simulink model "acc_with_sensor"  (R2021b)
settings: Solver=FixedStepAuto  StartTime=0.0  StopTime=206  FixedStep=0.0005  RelTol=1e-3
InitFcn:
  | G=9.81;
  | m=1660;
  | rw=0.325;
  | Caf=74070;
  | Car=58525;
  | Iz=2778.5;
  | d = 1.502;
  | lf =1.1135;
  | lr =1.5065;
  | L = 2.62;
  | kph2mps=1/3.6;
values from neighbouring files (symbols this model uses):
  Leftdis_PV_switch = 2    [acc_plot_backup.m]
  s_path = [0 1.10508939428 2.2141958029 3.32141571172 4.42705301151 5.53154548532 6.63517443471 7.73808041313 8.84055018688 9.94289959674 11.0453539299 12.1480581097 ... (1001 elements, 1001x1)]    [200_100radius.mat]    (also in LV_Clothoid_S_Turn_path.mat = [0 0.966832089581 1.93621320584 2.90214024471 3.86476766313 ; NEDC_path.mat = [0 0.414605943146 0.832514087334 1.25401518562 1.68216660344; Straight_East_into_curve.mat = [0 1.65770560069 3.32192925577 4.98420060507 6.64484613518 8; acc_plot_backup.m = Station_HV_m)
  X_path = [0 1.10508939428 2.2141958029 3.32141571172 4.42705301151 5.53154548532 6.63517443471 7.73808041313 8.84055018688 9.94289959674 11.0453539299 12.1480581097 ... (1001 elements, 1001x1)]    [200_100radius.mat]    (also in LV_Clothoid_S_Turn_path.mat = [-10 -9.03316791042 -8.06378679416 -7.09785975529 -6.1352323; NEDC_path.mat = [0 0.414605943146 0.832514087334 1.25401518562 1.68216660344; Straight_East_into_curve.mat = [0 1.65770560069 3.32192925577 4.98420060507 6.64484613518 8; acc_plot_backup.m = X_HV_m)
  Y_path = [0 -1.70364610795e-18 -7.41532896709e-18 1.46822109542e-17 4.74557362791e-17 6.12980216762e-17 9.25043977736e-17 1.24088240159e-16 1.5099156923e-16 1.7058517853e-16 1.90629227614e-16 2.09673434424e-16 ... (1001 elements, 1001x1)]    [200_100radius.mat]    (also in LV_Clothoid_S_Turn_path.mat = [0 -8.46153035536e-19 5.07382551045e-18 2.07356032218e-17 3.; NEDC_path.mat = [0 -3.50680326162e-18 -2.14111304971e-18 3.38197671014e-18 3; Straight_East_into_curve.mat = [0 1.29197709199e-18 2.81882429322e-18 3.49020462564e-17 6.7; acc_plot_backup.m = Y_HV_m)
undefined symbols (not defined in the file or in its folder): C_TICK_TIME_S, Cut_in_Secenary_flg, ENUM_ACCSTATE_DISABLED, ENUM_ACCSTATE_OFF, ENUM_ACCSTATE_STANDBY, FALSE, KVDI_ACCLongPressTime_ms, KVDI_ACCMaxActSpeed_kph, KVDI_ACCSetSpdIntial_kph, KVDI_ACCSpdLargeChange_kph, KVDI_LongPressConTime_ms, ONE_FLOAT, ONE_INT, raptor_xcp_function, T, TRUE, UseTTC_switch, ZERO_FLOAT, ZERO_INT
libraries: ADASLibrary x29, simulink x22, Raptor_lib x11, dspstat3 x6, simulink_extras x6, Solver_SF x1, mpclib x1
(part 1 of 9)
settings Model: Creator=power  LastModifiedBy=power
settings DataIOCC: ReturnWorkspaceOutputs=off

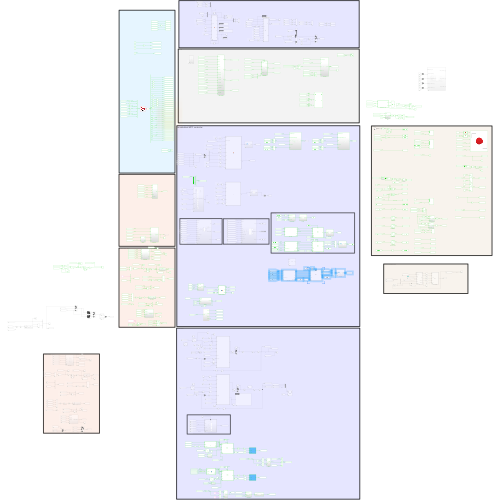
[thumbnail: Simulink's stored preview of the top-level diagram]
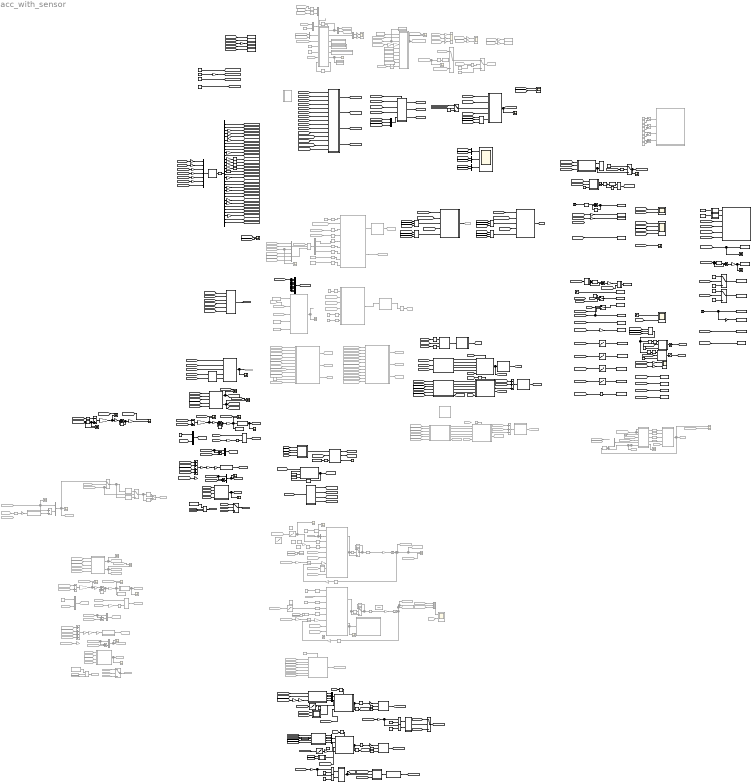
== system acc_with_sensor ==
  note: Combine_Version
  note: Combine_delta_u
  note: Combine_Version
  note: Constraint MPC TEST
  note: Lateral MPC controller
  note: Kalman Filter
  note: Carsim
  note: Record data
  note: Longitudinal MPC controller
  note: Camera_emulator
  note: Longitudinal Constraint MPC controller
  note: Doesn't work with low speed
  note: Estimator
  note: Car_following_trajectory_planning
  note: Car_following_trajectory_planning
  1-D Lookup Table Accel Limit1 : Lookup_n-D  NumberOfTableDimensions=1  BreakpointsForDimension1=[0,5,20,30]  Table=[4,4,2,2]  InternalRulePriority=Speed  RndMeth=Simplest  InputSameDT=on
  1-D Lookup Table Deccel Limit2 : Lookup_n-D  NumberOfTableDimensions=1  BreakpointsForDimension1=[0,5,20,30]  Table=[-5,-5,-2.5,-2.5]  InternalRulePriority=Speed  RndMeth=Simplest  InputSameDT=on
  1-D Lookup Table Jerk LowLimit1 : Lookup_n-D  NumberOfTableDimensions=1  BreakpointsForDimension1=[0,5,20,30]  Table=[-5,-5,-2.5,-2.5]  InternalRulePriority=Speed  RndMeth=Simplest  InputSameDT=on
  1-D Lookup Table Jerk UpLimit1 : Lookup_n-D  NumberOfTableDimensions=1  BreakpointsForDimension1=[0,5,20,30]  Table=[5,5,2.5,2.5]  InternalRulePriority=Speed  RndMeth=Simplest  InputSameDT=on
  1-D Lookup Table1 : Lookup_n-D  Commented=on  NumberOfTableDimensions=1  BreakpointsForDimension1=[35 40 70 80]/3.6  Table=[0.01 0.01 0.0025 0.0025]  InternalRulePriority=Speed  RndMeth=Simplest  InputSameDT=on
  1-D Lookup Table2 : Lookup_n-D  Commented=on  NumberOfTableDimensions=1  BreakpointsForDimension1=[0 10 35 40]/3.6  Table=[0.25 0.25 0.025 0.025]  InternalRulePriority=Speed  RndMeth=Simplest  InputSameDT=on
  1-D Lookup Table6 : Lookup_n-D  Commented=on  NumberOfTableDimensions=1  BreakpointsForDimension1=[35 40 70 80]/3.6  Table=[0.01 0.01 0.0025 0.0025]  InternalRulePriority=Speed  RndMeth=Simplest  InputSameDT=on
  1-D Lookup Table7 : Lookup_n-D  NumberOfTableDimensions=1  BreakpointsForDimension1=[35 40 70 80]/3.6  Table=[0.01 0.01 0.0025 0.0025]  InternalRulePriority=Speed  RndMeth=Simplest  InputSameDT=on
  1-D Lookup Table8 : Lookup_n-D  NumberOfTableDimensions=1  BreakpointsForDimension1=[0 10 35 40]/3.6  Table=[0.25 0.25 0.025 0.025]  InternalRulePriority=Speed  RndMeth=Simplest  InputSameDT=on
  11:20 : Selector  Commented=on  InputPortWidth=20  IndexOptions=Index vector (dialog)  Indices=[11:20]  OutputSizes=1
  1:10 : Selector  Commented=on  InputPortWidth=20  IndexOptions=Index vector (dialog)  Indices=[1:10]  OutputSizes=1
  ACCSpdCalculation : Subsystem  Commented=on
  ACC_Mode_Selector : Subsystem
  ACC_Mode_Selector3 : Subsystem
  Abs : Abs
  Abs2 : Abs
  Abs4 : Abs
  Abs6 : Abs  Commented=on
  Acceleration controller2 : MATLAB Function  TreatAsAtomicUnit=on
  Add Constant : Bias  Bias=-2
  Add Constant4 : Bias  Bias=+2
  Add Constant5 : Bias  Bias=-2
  Add1 : Sum  Commented=on  Inputs=++-
  Add{4,9..10,60} (4 alike) : Sum  Inputs=-+
  Add11 : Sum
  Add15 : Sum
  Add19 : Sum  Commented=on  Inputs=+-
  Add20 : Sum  Inputs=+-
  Add21 : Sum  Commented=on  Inputs=++++
  Add22 : Sum  Commented=on  Inputs=-+
  Add23 : Sum  Commented=on
  Add25 : Sum  Inputs=++-
  Add26 : Sum  Commented=on  Inputs=+-
  Add32 : Sum  Inputs=+-
  Add56 : Sum  Inputs=++++
  Add62 : Sum
  Add7 : Sum  Commented=on  Inputs=+-
  Bus Creator : BusCreator  Inputs=5
  Bus Creator1 : BusCreator  Inputs=5
  Camera : Subsystem
  CarSim S-Function : Solver_SF/CarSim S-Function  Priority=1  SIMFILE=simfile.sim  Run_RTs=off  vs_state_ind=Run  StopMode_ind=Vehicle Model
  Compare To Constant2 : simulink/Logic and Bit Operations/Compare To Constant  Commented=on  relop=>  const=.015  OutDataTypeStr=boolean
  Compare To Constant4 : simulink/Logic and Bit Operations/Compare To Constant  relop===  const=0  OutDataTypeStr=boolean
  Compare To Constant5 : simulink/Logic and Bit Operations/Compare To Constant  relop=>=  const=2  OutDataTypeStr=boolean
  Compare To Zero : simulink/Logic and Bit Operations/Compare To Zero  relop===  OutDataTypeStr=boolean
  Compare To Zero1 : simulink/Logic and Bit Operations/Compare To Zero  relop=~=  OutDataTypeStr=boolean
  Constant : Constant  Value=0  SampleTime=T
  Constant1 : Constant  SampleTime=T
  Constant10 : Constant  Commented=on  Value=0.1
  Constant101 : Constant  Value=720  SampleTime=T
  Constant102 : Constant  Value=720  SampleTime=T
  Constant103 : Constant  Value=-720  SampleTime=T
  Constant{8,51,58,104} (4 alike) : Constant  Commented=on  SampleTime=T
  Constant105 : Constant  Value=-720  SampleTime=T
  Constant106 : Constant  Value=35  SampleTime=T
  Constant107 : Constant  Value=30  SampleTime=T
  Constant108 : Constant  Value=0.5  SampleTime=T
  Constant11 : Constant  Value=60  SampleTime=T
  Constant{12..13,24,45} (4 alike) : Constant  Commented=on  OutDataTypeStr=boolean
  Constant14 : Constant  Value=1270+22*4+88.6+54.4  SampleTime=T
  Constant{15,39,46..47} (4 alike) : Constant  Commented=on  Value=0  OutDataTypeStr=boolean
  Constant{3,9,16,28,92} (5 alike) : Constant  Commented=on
  Constant17 : Constant  Commented=on  Value=0.3
  Constant18 : Constant  Commented=on  Value=0.025
  Constant19 : Constant  SampleTime=T
  Constant2 : Constant  Commented=on  Value=2
  Constant20 : Constant  Value=10  SampleTime=T
  Constant21 : Constant  Value=10  SampleTime=T
  Constant{7,22..23,29} (4 alike) : Constant  Value=1.5  SampleTime=T
  Constant26 : Constant  Value=X_path  SampleTime=T
  Constant27 : Constant  Value=Y_path  SampleTime=T
  Constant30 : Constant  Value=35
  Constant31 : Constant  Value=3  SampleTime=T
  Constant32 : Constant  Value=30
  Constant33 : Constant  Value=5  SampleTime=T
  Constant34 : Constant  Value=-3  SampleTime=T
  Constant35 : Constant  Value=-5  SampleTime=T
  Constant38 : Constant  Commented=on  Value=0
  Constant4 : Constant  Commented=on  Value=0.0025
  Constant40 : Constant  Commented=on  Value=0.2
  Constant41 : Constant  Commented=on  Value=0.2
  Constant42 : Constant  Commented=on  Value=7
  Constant43 : Constant  Commented=on  Value=0.0125
  Constant44 : Constant  Commented=on  Value=100
  Constant48 : Constant  Commented=on  Value=75
  Constant5 : Constant  Commented=on  Value=0.2
  Constant50 : Constant  Commented=on  Value=3
  Constant52 : Constant  Commented=on  Value=1.015
  Constant54 : Constant  Commented=on  Value=2.910-1.015
  Constant55 : Constant  Commented=on  Value=1270+22*4+88.6+54.4
  Constant56 : Constant  Commented=on  Value=0.1
  Constant57 : Constant  Commented=on  Value=73922.12
  Constant59 : Constant  Commented=on  Value=54682
  Constant6 : Constant  Commented=on  Value=2.5
  Constant60 : Constant  Commented=on  Value=15/3.6
  Constant61 : Constant  Commented=on  Value=0
  Constant62 : Constant  Value=Leftdis_PV_switch
  Constant63 : Constant  Value=0
  Constant67 : Constant  SampleTime=T
  Constant83 : Constant  Value=0.3  SampleTime=T
  Constant84 : Constant  Value=0.1  SampleTime=T
  Constant85 : Constant  Commented=on  OutDataTypeStr=boolean  SampleTime=T
  Constant98 : Constant  Commented=on  Value=Leftdis_PV_switch
  Constant99 : Constant  Commented=on  Value=0
  Cos : Trigonometry  Operator=tan
  Cos1 : Trigonometry  Commented=on  Operator=tan
  Cut-in strategy : Subsystem
  Delay : Delay  DelayLength=1  SampleTime=T
  Delay{1,16..19,50} (6 alike) : Delay  DelayLength=1
  Delay10 : Delay  Commented=on  DelayLength=1  InitialConditionSource=Input port  InitialCondition=[50/3.6 0]'  SampleTime=T
      settings: InputPortMap=u0,p4
  Delay11 : Delay  DelayLength=1  SampleTime=T
  Delay14 : Delay  Commented=on  DelayLength=1
  Delay2 : Delay  DelayLength=1  InitialConditionSource=Input port  SampleTime=T
      settings: InputPortMap=u0,p4
  Delay3 : Delay  DelayLength=1  SampleTime=T
  Delay4 : Delay  Commented=on  DelayLength=1  SampleTime=T
  Delay48 : Delay  Commented=on  DelayLength=1  InitialCondition=[1 0;0 1]  SampleTime=T
  Delay49 : Delay  Commented=on  DelayLength=1  InitialConditionSource=Input port  InitialCondition=[50/3.6 0]'  SampleTime=T
      settings: InputPortMap=u0,p4
  Delay6 : Delay  DelayLength=1  InitialConditionSource=Input port  SampleTime=T
      settings: InputPortMap=u0,p4
  Delay7 : Delay  Commented=on  DelayLength=1  SampleTime=T
  Delay8 : Delay  Commented=on  DelayLength=1  SampleTime=T
  Demux : Demux  Outputs=32
  Demux2 : Demux  Commented=on  Outputs=[10]
  Demux3 : Demux  Commented=on  Outputs=3
  Demux6 : Demux  Commented=on  Outputs=2
  Demux8 : Demux  Commented=on  Outputs=2
  Detect Increase : simulink/Logic and Bit Operations/Detect Increase  vinit=0.0  OutDataTypeStr=boolean
  Display{,1,4..7} (6 alike) : Display  Commented=on
      Display4 settings: Format=bank
      Display5 settings: Format=bank
      Display6 settings: Format=bank
      Display7 settings: Format=bank
  Dynamic_Model : MATLAB Function  TreatAsAtomicUnit=on
  Estimation_TTCx_PV2 : MATLAB Function  TreatAsAtomicUnit=on
  From10 : From  Commented=on  GotoTag=Est_switch
  From{103,138,159,186,190,510} (6 alike) : From  Commented=on  GotoTag=ACCSetSpeed_mps
  From121 : From  Commented=on  GotoTag=Acc_Mode
  From{124,185,212,508} (4 alike) : From  Commented=on  GotoTag=RR_new
  From126 : From  Commented=on  GotoTag=Steer_Dynamic_deg
  From{127,216..217,241,402,447} (6 alike) : From  Commented=on  GotoTag=Yaw_rate_radps
  From{25,128,162,174,221,399} (6 alike) : From  Commented=on  GotoTag=Steer_SW_deg
  From129 : From  Commented=on  GotoTag=y_ref
  From{16,18,24,33,80,92,132,154,160,164,169,176,191,237,247..248,253,396,435,511} (20 alike) : From  Commented=on  GotoTag=Vx_HV_mps
  From134 : From  Commented=on  GotoTag=Acc_Mode
  From{49,135,200,515} (4 alike) : From  Commented=on  GotoTag=RVx
  From{50,137,141,268,516} (5 alike) : From  Commented=on  GotoTag=RAx
  From{17,37,139..140,149,155,161,177,199,243,401,514} (12 alike) : From  Commented=on  GotoTag=Ax_HV_mps2
  From142 : From  Commented=on  GotoTag=ax
  From{153,166,180,232,238,403} (6 alike) : From  Commented=on  GotoTag=Vy_HV_mps
  From{21,55,157,517} (4 alike) : From  Commented=on  GotoTag=Vx_p
  From163 : From  Commented=on  GotoTag=RR
  From{167,219,234,258,273} (5 alike) : From  Commented=on  GotoTag=Vy_e_output
  From{170,214,398,433} (4 alike) : From  Commented=on  GotoTag=LaneAvail_flg
  From173 : From  Commented=on  GotoTag=y_ref
  From{175,193,434,456} (4 alike) : From  Commented=on  GotoTag=Ry
  From181 : From  Commented=on  GotoTag=Est_switch
  From187 : From  Commented=on  GotoTag=RR_est
  From188 : From  Commented=on  GotoTag=x_translate
  From192 : From  Commented=on  GotoTag=RV_est
  From195 : From  Commented=on  GotoTag=RA_est
  From23 : From  Commented=on  GotoTag=LFC_Mode
  From233 : From  Commented=on  GotoTag=Ay_HV_mps2
  From239 : From  Commented=on  GotoTag=Estimated_Vx_mps
  From242 : From  Commented=on  GotoTag=Vy_e_Small_YawRate
  From244 : From  Commented=on  GotoTag=Vy_e_Small_YawRate
  From245 : From  Commented=on  GotoTag=ax_c_old
  From246 : From  Commented=on  GotoTag=Ay_HV_mps2
  From255 : From  Commented=on  GotoTag=Estimated_Vy_mps
  From257 : From  Commented=on  GotoTag=Estimated_Vy_mps
  From31 : From  Commented=on  GotoTag=RR_est
  From38 : From  Commented=on  GotoTag=RV_est
  From39 : From  Commented=on  GotoTag=RA_est
  From397 : From  Commented=on  GotoTag=y_ref
  From429 : From  Commented=on  GotoTag=LeftDis_Camera
  From430 : From  Commented=on  GotoTag=LeftDis_PV
  From431 : From  Commented=on  GotoTag=delta_yaw
  From432 : From  Commented=on  GotoTag=Rx
  From436 : From  Commented=on  GotoTag=delta_x_19
  From437 : From  Commented=on  GotoTag=LeftDis_PV_one
  From438 : From  Commented=on  GotoTag=LeftDis_PV_multi
  From439 : From  Commented=on  GotoTag=Roll_rate_L1_radps
  From440 : From  Commented=on  GotoTag=delta_yaw
  From441 : From  Commented=on  GotoTag=X_HV_m
  From442 : From  Commented=on  GotoTag=delta_y_19
  From443 : From  Commented=on  GotoTag=Y_HV_m
  From444 : From  Commented=on  GotoTag=Yaw_HV_deg
  From445 : From  Commented=on  GotoTag=delta_x_19
  From446 : From  Commented=on  GotoTag=Yaw_HV_deg
  From448 : From  Commented=on  GotoTag=X_PV_m
  From449 : From  Commented=on  GotoTag=Y_PV_m
  From450 : From  Commented=on  GotoTag=Roll_rate_L2_radps
  From451 : From  Commented=on  GotoTag=y_translate
  From452 : From  Commented=on  GotoTag=Roll_rate_R1_radps
  From453 : From  Commented=on  GotoTag=Roll_rate_R2_radps
  From454 : From  Commented=on  GotoTag=x_translate
  From455 : From  Commented=on  GotoTag=yaw_rotate
  From457 : From  Commented=on  GotoTag=Roll_rate_L1_radps
  From458 : From  Commented=on  GotoTag=Roll_rate_R1_radps
  From459 : From  Commented=on  GotoTag=sensor_dectect_y_m
  From507 : From  Commented=on  GotoTag=Est_switch
  From509 : From  Commented=on  GotoTag=RR_est
  From512 : From  Commented=on  GotoTag=RV_est
  From513 : From  Commented=on  GotoTag=RA_est
  Gain : Gain  Gain=0.25
  Gain{1,9..10,15,47..49,58} (8 alike) : Gain  Gain=1/3.6
  Gain12 : Gain  Gain=0.5
  Gain{8,13,19..21,31..32,78} (8 alike) : Gain  Gain=3.6
  Gain{14,27,44,71} (4 alike) : Gain  Commented=on  Gain=pi/180
  Gain2 : Gain  Commented=on  Gain=1.5
  Gain22 : Gain  Gain=0.5
  Gain23 : Gain  Commented=on  Gain=20
  Gain{24..26,34,41} (5 alike) : Gain  Commented=on  Gain=1/20
  Gain28 : Gain  Commented=on  Gain=20
  Gain3 : Gain  Gain=9.81
  Gain30 : Gain  Gain=pi/180
  Gain{33,36..38} (4 alike) : Gain
  Gain35 : Gain  Gain=-1
  Gain4 : Gain  Gain=9.81
  Gain{40,43,51..55,80..81} (9 alike) : Gain  Commented=on  Gain=3.6
  Gain42 : Gain  Gain=pi/180
  Gain45 : Gain  Gain=0.1
  Gain46 : Gain  Commented=on  Gain=0.1
  Gain5 : Gain  Gain=180/pi
  Gain50 : Gain  Gain=9.81
  Gain56 : Gain  Gain=0.1
  Gain{57,59..61} (4 alike) : Gain  Gain=pi/30
  Gain6 : Gain  Gain=100
  Gain70 : Gain  Commented=on  Gain=0.25
  Gain72 : Gain  Gain=180/pi
  Gain73 : Gain  Commented=on  Gain=0.1
  Gain74 : Gain  Commented=on  Gain=0.1
  Gain75 : Gain  Commented=on  Gain=180/pi
  Gain77 : Gain  Gain=20
  Gain79 : Gain  Gain=pi/180
  Gain82 : Gain  Gain=1/20
  Gain83 : Gain  Gain=20
  Goto126 : Goto  Commented=on  GotoTag=Steer_IN_deg
  Goto127 : Goto  Commented=on  GotoTag=Steer_Dynamic_deg0  TagVisibility=global
  Goto128 : Goto  Commented=on  GotoTag=Steer_Kinematic_deg0  TagVisibility=global
  Goto133 : Goto  Commented=on  GotoTag=delta_yaw
  Goto134 : Goto  Commented=on  GotoTag=delta_y_19
  Goto135 : Goto  Commented=on  GotoTag=y_ref
  Goto136 : Goto  Commented=on  GotoTag=LeftDis_PV
  Goto137 : Goto  Commented=on  GotoTag=LeftDis_PV_one
  Goto138 : Goto  Commented=on  GotoTag=Rx
  Goto139 : Goto  Commented=on  GotoTag=Ry
  Goto140 : Goto  Commented=on  GotoTag=x_translate
  Goto141 : Goto  Commented=on  GotoTag=yaw_rotate
  Goto142 : Goto  Commented=on  GotoTag=LeftDis_PV_multi
  Goto143 : Goto  Commented=on  GotoTag=y_translate
  Goto144 : Goto  Commented=on  GotoTag=delta_x_19
  Goto{22,39,54,152} (4 alike) : Goto  Commented=on  GotoTag=th_acc
  Goto{28,40,50,153} (4 alike) : Goto  Commented=on  GotoTag=Desired_distance
  Goto{24,41,44,155} (4 alike) : Goto  Commented=on  GotoTag=spd_acc
  Goto19 : Goto  Commented=on  GotoTag=Steer_Kinematic_deg
  Goto30 : Goto  Commented=on  GotoTag=Acc_Mode
  Goto31 : Goto  Commented=on  GotoTag=ax_c_old
  Goto38 : Goto  Commented=on  GotoTag=Steer_Dynamic_deg
  Goto49 : Goto  Commented=on  GotoTag=Estimated_Vx_mps
  Goto58 : Goto  Commented=on  GotoTag=delta_u_TH
  Goto84 : Goto  Commented=on  GotoTag=Estimated_Vy_mps
  Goto90 : Goto  Commented=on  GotoTag=Vy_e_Small_YawRate
  Goto91 : Goto  Commented=on  GotoTag=Vy_e_output
  Goto93 : Goto  Commented=on  GotoTag=LeftDis_PV_multi
  Goto95 : Goto  Commented=on  GotoTag=y_translate
  IC : InitialCondition  Commented=on  Value=0
  Kalman_Filter_LatSpd1 : MATLAB Function  Commented=on  TreatAsAtomicUnit=on
  Kinematic_Model : MATLAB Function  TreatAsAtomicUnit=on
  Latch : Subsystem
  Latch2 : Subsystem
  LateralMotionKF1 : MATLAB Function  Commented=on  TreatAsAtomicUnit=on
  Limit : ADASLibrary/Limit  SystemSampleTime=-1  VariantActivationTime=update diagram  Latency=0  AutoFrameSizeCalculation=off
      settings: SourceProductName=ADASLibrary
  Limit1 : ADASLibrary/Limit  SystemSampleTime=-1  VariantActivationTime=update diagram  Latency=0  AutoFrameSizeCalculation=off
      settings: SourceProductName=ADASLibrary
  Logical Operator : Logic  Operator=NOT  AllPortsSameDT=off  OutDataTypeStr=boolean
  Logical Operator1 : Logic  Operator=NOT  AllPortsSameDT=off  OutDataTypeStr=boolean
  Logical Operator2 : Logic  Commented=on  Operator=NOT  AllPortsSameDT=off  OutDataTypeStr=boolean
  Logical Operator3 : Logic  AllPortsSameDT=off  OutDataTypeStr=boolean
  MATLAB Function1 : MATLAB Function  Commented=on  TreatAsAtomicUnit=on
  MATLAB Function13 : MATLAB Function  TreatAsAtomicUnit=on
  MATLAB Function17 : MATLAB Function  Commented=on  TreatAsAtomicUnit=on
  MATLAB Function5 : MATLAB Function  TreatAsAtomicUnit=on
  MPC : MATLAB Function  Commented=on  TreatAsAtomicUnit=on
  MPC Controller : mpclib/MPC Controller  Commented=on  SCDEnableBlockLinearizationSpecification=on  is_multiple=0  enable_value=0  return_u0=off  updateMPCinCallerWorkspace=on  md_inport=on  mv_inport=off  uref_inport=off  return_cost=off  return_mvseq=off  return_qpstatus=off  return_xseq=off  return_state=off  return_ovseq=off  state_inport=on  umin_inport=off  umax_inport=off  ymin_inport=off  ymax_inport=off  cc_inport=off  ywt_inport=off  uwt_inport=off  duwt_inport=off  rhoeps_inport=off  pm_inport=off  MaximumP=10  HorizonChoice=FixedHorizon  n_ts=0.1  n_p=10  n_mv=1  n_md=1  n_ud=0  n_mo=1  n_uo=0  BlockDataType=double  SampleTimeInherited=off  switch_inport=off
  MPC_ACC : MATLAB Function  Commented=on  TreatAsAtomicUnit=on
  MPC_ACC1 : MATLAB Function  Commented=on  TreatAsAtomicUnit=on
  MPC_ACC4 : MATLAB Function  TreatAsAtomicUnit=on
  MPC_ACC5 : MATLAB Function  TreatAsAtomicUnit=on
  MPC_Bicycle_LDC1 : MATLAB Function  Commented=on  TreatAsAtomicUnit=on
  Manual Switch{,1,5,9,11..12} (6 alike) : ManualSwitch  Commented=on
  Manual Switch10 : ManualSwitch  Commented=on  CurrentSetting=0
  Min : MinMax  Inputs=2
  Multiport Switch{,1,3..4,13..14} (6 alike) : MultiPortSwitch  DataPortOrder=Zero-based contiguous  Inputs=2  DiagnosticForDefault=None  zeroidx=on
  Multiport Switch10 : MultiPortSwitch  Commented=on  Inputs=2
  Multiport Switch2 : MultiPortSwitch  Commented=on  DataPortOrder=Zero-based contiguous  Inputs=2  DiagnosticForDefault=None  zeroidx=on
  Multiport Switch5 : MultiPortSwitch  Inputs=2
  Mux : Mux  Inputs=7
  Mux1 : Mux  Inputs=2
  Mux10 : Mux  Commented=on  Inputs=2
  Mux11 : Mux  Commented=on  Inputs=2
  Mux14 : Mux  Inputs=[1 9]
  Mux{15,23..25} (4 alike) : Mux  Commented=on  Inputs=[1 19]
  Mux16 : Mux  Inputs=[1 9]
  Mux17 : Mux  Commented=on  Inputs=2
  Mux2 : Mux  Inputs=2
  Mux20 : Mux  Inputs=[1 9]
  Mux3 : Mux  Inputs=2
  Mux4 : Mux  Inputs=3
  Mux5 : Mux  Inputs=10
  Mux6 : Mux  Commented=on  Inputs=3
  Mux7 : Mux  Commented=on  Inputs=3
  Mux8 : Mux  Commented=on  Inputs=3
  Mux9 : Mux  Commented=on  Inputs=[3 1 1 1]
  Old_Relative_Dynamic : Subsystem  Commented=on
  PV_trajectory_planning : Subsystem
  PV_trajectory_planning1 : Subsystem  Commented=on
  Product2 : Product
  Product3 : Product  Commented=on
  QP_logitudinal1 : MATLAB Function  Commented=on  TreatAsAtomicUnit=on
  Quantizer{1..6} (6 alike) : Quantizer  QuantizationInterval=0.02
  R selector : Subsystem  Commented=on
  R selector1 : Subsystem  Commented=on
  R selector4 : Subsystem
  R selector5 : Subsystem
  Radians to Degrees1 : simulink_extras/Transformations/Radians to Degrees  Commented=on
  Radians to Degrees2 : simulink_extras/Transformations/Radians to Degrees  Commented=on
  Radians to Degrees5 : simulink_extras/Transformations/Radians to Degrees
  Radians to Degrees6 : simulink_extras/Transformations/Radians to Degrees
  Relational Operator : RelationalOperator  OutDataTypeStr=boolean  RndMeth=Simplest
  Relational Operator1 : RelationalOperator  Operator=<=  OutDataTypeStr=boolean  RndMeth=Simplest
  Relational Operator10 : RelationalOperator  Operator=<=  OutDataTypeStr=boolean  RndMeth=Simplest
  Relational Operator2 : RelationalOperator  Commented=on  Operator=isNaN  OutDataTypeStr=boolean  RndMeth=Simplest
  Relational Operator3 : RelationalOperator  Commented=on  OutDataTypeStr=boolean  RndMeth=Simplest
  Relational Operator4 : RelationalOperator  Commented=on  Operator=isNaN  OutDataTypeStr=boolean  RndMeth=Simplest
  Relational Operator9 : RelationalOperator  OutDataTypeStr=boolean  RndMeth=Simplest
  Relative_Dynamic : Subsystem
  Reshape : Reshape  Commented=on
  Saturation : Saturate  UpperLimit=100  LowerLimit=-100
  Saturation1 : Saturate  UpperLimit=10  LowerLimit=0
  Saturation2 : Saturate  Commented=on  UpperLimit=30/3.6  LowerLimit=5/3.6
  Saturation3 : Saturate  Commented=on  UpperLimit=720  LowerLimit=-720
  Saturation4 : Saturate  Commented=on  UpperLimit=720  LowerLimit=-720
  Saturation7 : Saturate  UpperLimit=10  LowerLimit=0
  Scope{,3..4,23,30,36,38,41,76,84,88..89,92} (13 alike) : Scope  Commented=on
  Scope{1,21,25,50,86..87,90..91} (8 alike) : Scope  Commented=on  NumInputPorts=2
  Scope{6..7,9..10,24,32,56,58,85,159} (10 alike) : Scope
  Scope11 : Scope  NumInputPorts=3
  Scope12 : Scope  NumInputPorts=4
  Scope{2,5,13,16,18,33,70..72,75,77..78} (12 alike) : Scope  NumInputPorts=2
  Smooth Switch : Subsystem
  Smooth Switch1 : Subsystem
  Smooth Switch4 : Subsystem
  Steer_Dynamic : Subsystem  mask{T=T, Np=10, Nc=3}
      mask prompts: T "Sample time"
      mask Display:
      | fprintf('MPC \n\n')
      | 
      | fprintf(['T=' num2str(T)])
  Steer_Kinematic : Subsystem  mask{T=T, Np=10, Nc=3}
      mask prompts: T "Sample time"
      mask help: Model : A,B,C,Yref,x_state
      mask Display:
      | fprintf('MPC \n\n')
      | 
      | fprintf(['T=' num2str(T)])
  Step : Step  Time=0  Before=1.5  After=1.5  SampleTime=T
  Step1 : Step  Time=0  Before=1.5  After=1.5  SampleTime=T
  Step2 : Step  Time=0  After=0.1  SampleTime=0
  Step3 : Step  Time=0  Before=5  After=5  SampleTime=T
  Subsystem : Subsystem  Commented=on
  Subsystem1 : Subsystem  Commented=on
  Subsystem17 : Subsystem
  Subsystem2 : Subsystem
  Subsystem21 : Subsystem  mask{T=T, Np=10, Nc=3, Q=1, R=0.2}
      mask prompts: T "Sample time"
      mask Display:
      | fprintf('MPC \n\n')
      | 
      | fprintf(['T=' num2str(T)])
  Subsystem22 : Subsystem  Commented=on
  Subsystem23 : Subsystem  mask{T=T, Np=10, Nc=3, Q=1, R=0.2}
      mask prompts: T "Sample time"
      mask Display:
      | fprintf('MPC \n\n')
      | 
      | fprintf(['T=' num2str(T)])
  Subsystem25 : Subsystem
  Subsystem3 : Subsystem
  Subsystem4 : Subsystem
  Subsystem5 : Subsystem  Commented=on
  Subsystem6 : Subsystem  Commented=on
  Subsystem7 : Subsystem  Commented=on  mask{T=T, Np=10, Nc=3, Q=1, R=0.2}
      mask prompts: T "Sample time"
      mask Display:
      | fprintf('MPC \n\n')
      | 
      | fprintf(['T=' num2str(T)])
  Subsystem8 : Subsystem  Commented=on
  Switch : Switch  Commented=on  Criteria=u2 > Threshold
  Switch{1,8,11..13,16} (6 alike) : Switch  Criteria=u2 ~= 0
  Switch10 : Switch  Commented=on
  Switch15 : Switch  Commented=on  Criteria=u2 ~= 0
  Switch2 : Switch  Commented=on  Criteria=u2 ~= 0
  Switch3 : Switch  Commented=on  Criteria=u2 > Threshold
  Switch4 : Switch  Commented=on  Criteria=u2 > Threshold
  Switch5 : Switch  Threshold=8
  Switch6 : Switch  Threshold=8
  Switch9 : Switch  Commented=on
  T : Gain  Gain=0.1
  T1 : Gain  Gain=0.1
  T2 : Gain  Commented=on  Gain=0.1
  To Workspace : ToWorkspace  VariableName=X_HV_m  SampleTime=-1
  To Workspace1 : ToWorkspace  VariableName=Y_HV_m  SampleTime=-1
  To Workspace10 : ToWorkspace  VariableName=TH  SampleTime=-1
  To Workspace11 : ToWorkspace  VariableName=RR  SampleTime=-1
  To Workspace12 : ToWorkspace  VariableName=Desired_distance  SampleTime=-1
  To Workspace13 : ToWorkspace  VariableName=C_tick_time  SampleTime=-1
  To Workspace14 : ToWorkspace  VariableName=Ax_HV_mps2  SampleTime=-1
  To Workspace15 : ToWorkspace  VariableName=V_ref_kph  SampleTime=-1
  To Workspace16 : ToWorkspace  VariableName=Ax_Up_Limit  SampleTime=-1
  To Workspace17 : ToWorkspace  VariableName=Ax_Low_Limit  SampleTime=-1
  To Workspace18 : ToWorkspace  VariableName=Jerk_x_Up_Limit  SampleTime=-1
  To Workspace19 : ToWorkspace  VariableName=Jerk_x_Low_Limit  SampleTime=-1
  To Workspace2 : ToWorkspace  VariableName=Yaw_HV_deg  SampleTime=-1
  To Workspace20 : ToWorkspace  VariableName=Acc_Mode  SampleTime=-1
  To Workspace21 : ToWorkspace  VariableName=Ay_Low_Limit  SampleTime=-1
  To Workspace22 : ToWorkspace  VariableName=Jerk_y_Up_Limit  SampleTime=-1
  To Workspace23 : ToWorkspace  VariableName=Jerk_y_Low_Limit  SampleTime=-1
  To Workspace24 : ToWorkspace  VariableName=Ay_HV_mps2  SampleTime=-1
  To Workspace25 : ToWorkspace  VariableName=y_error  SampleTime=-1
  To Workspace26 : ToWorkspace  VariableName=Steer_SW_deg  SampleTime=-1
  To Workspace27 : ToWorkspace  Commented=on  VariableName=Yaw_Est_deg1  SampleTime=-1
  To Workspace29 : ToWorkspace  VariableName=TTC  SampleTime=-1
  To Workspace3 : ToWorkspace  VariableName=Station_HV_m  SampleTime=-1
  To Workspace30 : ToWorkspace  VariableName=X_APV_m  SampleTime=T
  To Workspace31 : ToWorkspace  VariableName=Y_APV_m  SampleTime=T
  To Workspace32 : ToWorkspace  VariableName=APV_kph  SampleTime=T
  To Workspace34 : ToWorkspace  VariableName=Ax_APV_mps2  SampleTime=T
  To Workspace36 : ToWorkspace  VariableName=Station_APV_m  SampleTime=T
  To Workspace4 : ToWorkspace  VariableName=Jerk_y  SampleTime=-1
  To Workspace40 : ToWorkspace  VariableName=Yaw_Est_deg  SampleTime=-1
  To Workspace42 : ToWorkspace  Commented=on  VariableName=Vy_HV_kph  SampleTime=-1
  To Workspace43 : ToWorkspace  Commented=on  VariableName=Vy_e_output  SampleTime=-1
  To Workspace5 : ToWorkspace  VariableName=Ay_Up_Limit  SampleTime=-1
  To Workspace6 : ToWorkspace  VariableName=HV_kph  SampleTime=-1
  To Workspace7 : ToWorkspace  VariableName=PV_kph  SampleTime=-1
  To Workspace8 : ToWorkspace  VariableName=Jerk_x  SampleTime=-1
  To Workspace9 : ToWorkspace  VariableName=TH_ref  SampleTime=T
  Transfer Fcn3 : TransferFcn  Commented=on  Denominator=[0.3 1]
  Unit Delay : UnitDelay  Commented=on  SampleTime=-1  HasFrameUpgradeWarning=on
  Unit Delay2 : UnitDelay  Commented=on  SampleTime=-1  HasFrameUpgradeWarning=on
  Unit Delay4 : UnitDelay  Commented=on  SampleTime=T  HasFrameUpgradeWarning=on
  Unit Delay5 : UnitDelay  Commented=on  SampleTime=T  HasFrameUpgradeWarning=on
  V_rel Estimation : Subsystem
  Vx4 : Scope  Commented=on  NumInputPorts=3
  Vx5 : Scope  Commented=on  NumInputPorts=2
  Vx6 : Scope  Commented=on  NumInputPorts=2
  XY Graph : Record  FileSettingsInternal="{\"entries\":[{\"content\":{\"excelSettings\":{\"content\":{},\"type\":\"Streamout.ExcelSettings\"}},\"type\":\"Streamout.FileSettingStorage\",\"uuid\":\"f5793b5c-17c1-4d80-b906-8d311fc573b8\"}],\"packageUris\":[\"http://schema.mathworks.com/mf0/streamout_blocks/R2020a\"],\"version\":\"1.0\"}"  Layout=[1 1]  SignalsInternal="{\"entries\":[{\"content\":{\"signals\":[{\"content\":{\"blockPath\":[\"acc_with_sensor/XY Graph\"],\"channel\":[],\"dimensions\":[1],\"domain\":\"acc_with_sensor/XY Graph\",\"lineColor\":\"#a2142f\",\"plots\":[1],\"port\":1,\"sid\":[\"\"],\"signalID\":15776,\"signalName\":\"x\"},\"type\":\"RecordBlkView.Signal\",\"uuid\":\"b27bd53d-0975-41da-9d03-26616bef724a\"},{\"content\":{\"blockPath\":[\"acc_with_sensor/XY Graph\"],\"channel\":[],\"dimensions\":[1],\"domain\":\"acc_with_sensor/XY Graph\",\"lineColor\":\"#139fff\",\"plots\":[1],\"port\":2,\"sid\":[\"\"],\"signalID\":15780,\"signalName\":\"y\"},\"type\":\"RecordBlkView.Signal\",\"uuid\":\"106bb7c1-3890-427b-aa74-69dea0cde94a\"},{\"content\":{\"blockPath\":[\"acc_with_sensor/XY Graph\"],\"channel\":[],\"dimensions\":[1],\"domain\":\"acc_with_sensor/XY Graph\",\"lineColor\":\"#64d413\",\"plots\":[1],\"port\":3,\"sid\":[\"\"],\"signalID\":15784,\"signalName\":\"X_HV\"},\"type\":\"RecordBlkView.Signal\",\"uuid\":\"9e9f87ba-9ec3-4223-9e3a-e4abc68463f8\"},{\"content\":{\"blockPath\":[\"acc_with_sensor/XY Graph\"],\"channel\":[],\"dimensions\":[1],\"domain\":\"acc_with_sensor/XY Graph\",\"lineColor\":\"#ff13a6\",\"plots\":[1],\"port\":4,\"sid\":[\"\"],\"signalID\":15788,\"signalName\":\"Y_HV\"},\"type\":\"RecordBlkView.Signal\",\"uuid\":\"ebf38cc8-c54b-4403-87b1-8041da78f8fa\"},{\"content\":{\"blockPath\":[\"acc_with_sensor/XY Graph\"],\"channel\":[],\"dimensions\":[1],\"domain\":\"acc_with_sensor/XY Graph\",\"lineColor\":\"#ff6929\",\"plots\":[1],\"port\":5,\"sid\":[\"\"],\"signalID\":15792,\"signalName\":\"X_PV\"},\"type\":\"RecordBlkView.Signal\",\"uuid\":\"0d699c45-8040-4c97-a156-8ffb0b69b970\"},{\"content\":{\"blockPath\":[\"acc_with_sensor/XY Graph\"],\"channel\":[],\"dimensions\":[1],\"domain\":\"acc_with_sensor/XY Graph\",\"lineColor\":\"#b746ff\",\"plots\":[1],\"port\":6,\"sid\":[\"\"],\"signalID\":15796,\"signalName\":\"Y_PV\"},\"type\":\"RecordBlkView.Signal\",\"uuid\":\"8f872239-4f3e-42b3-82ae-4932be55b410\"}]},\"type\":\"RecordBlkView.InputSignals\",\"uuid\":\"5c4a2e27-ff75-4858-940e-dfe7bf690561\"}],\"packageUris\":[\"http://schema.mathworks.com/mf0/streamout_blocks/R2020a\"],\"version\":\"1.0\"}"  VisualizationBindings="{\"xyplotplugin\":{\"info\":[{\"series\":[{\"bindingParametersList\":[{\"parameter\":\"X-Axis\",\"signalID\":15776,\"signalName\":\"x\"},{\"parameter\":\"Y-Axis\",\"signalID\":15780,\"signalName\":\"y\"}],\"seriesID\":10259},{\"bindingParametersList\":[{\"parameter\":\"X-Axis\",\"signalID\":15784,\"signalName\":\"X_HV\"},{\"parameter\":\"Y-Axis\",\"signalID\":15788,\"signalName\":\"Y_HV\"}],\"seriesID\":4506},{\"bindingParametersList\":[{\"parameter\":\"X-Axis\",\"signalID\":15792,\"signalName\":\"X_PV\"},{\"parameter\":\"Y-Axis\",\"signalID\":15796,\"signalName\":\"Y_PV\"}],\"seriesID\":29876}],\"subplotID\":1}]}}"  CompatibilityTag=XY
  Zero-Order Hold{1..5,8..14,19..24,26..27,29,36} (22 alike) : ZeroOrderHold  Commented=on  SampleTime=T
  Zero-Order Hold17 : ZeroOrderHold  SampleTime=T
  Zero-Order Hold18 : ZeroOrderHold  SampleTime=T
  ascending : dspstat3/Sort  Commented=on  otype=Value  dir=Ascending  sortAlg=Quick sort  roundingMode=Floor  overflowMode=off  accumDataTypeStr=Inherit: Same as product output  accumLastDataTypeStr=Inherit: Same as product output
      settings: SourceProductBaseCode=DS
  cmd_limiter1 : Subsystem
  cmd_limiter11 : Subsystem
  cmd_limiter2 : Subsystem  Commented=on
  cmd_limiter3 : Subsystem  Commented=on
  cmd_limiter4 : Subsystem  Commented=on
  cmd_limiter9 : Subsystem
  descending : dspstat3/Sort  Commented=on  otype=Value  dir=Descending  sortAlg=Quick sort  roundingMode=Floor  overflowMode=off  accumDataTypeStr=Inherit: Same as product output  accumLastDataTypeStr=Inherit: Same as product output
      settings: SourceProductBaseCode=DS
  divide : Subsystem
  divide2 : Subsystem
  divide3 : Subsystem
  global to local1 : Subsystem  Commented=on
  global to local2 : Subsystem
  global to local3 : Subsystem
  preview : Subsystem
  r/l : Gain  Gain=0.33415/1.675
  r/l1 : Gain  Gain=0.33415/1.675
  r/l2 : Gain  Commented=on  Gain=0.33415/1.675
  record_delta_x : Subsystem
  record_delta_x1 : Subsystem  Commented=on
  record_delta_yaw : Subsystem
  record_delta_yaw1 : Subsystem  Commented=on
  rolling radius : Gain  Gain=0.325
  rolling radius1 : Gain  Commented=on  Gain=0.325
  rolling_avg1 : Subsystem
  sample time1 : Gain  Gain=1/0.1
  sample time2 : Gain  Gain=1/0.1
  way2 : Goto  Commented=on  GotoTag=LeftDis_Camera
  wires:
  Demux/1 -> [X_HV_m]
  CarSim S-Function/1 -> Zero-Order Hold18/1
  Demux/2 -> [Y_HV_m]
  Demux/3 -> Gain9/1
  Demux/4 -> Gain10/1
  Demux/5 -> Gain3/1
  Demux/6 -> Gain4/1
  Constant14/1 -> Zero-Order Hold17/1
  Subsystem2/4(Pb_RR) -> [Braking_Pressure_RR]
  [Driving_Brk_Cmd] -> Subsystem2/1(T_cmd)
  Subsystem2/1(Pb_LF) -> [Braking_Pressure_LF]
  Acceleration controller2/2(Tb) -> [Driving_Brk_Cmd]
  Acceleration controller2/3(Rtotal) -> Scope159/1
  Subsystem2/3(Pb_RL) -> [Braking_Pressure_RL]
  From37/1 -> Zero-Order Hold9/1
  From33/1 -> Zero-Order Hold8/1
  Acceleration controller2/1(Tr) -> [Driving_Torque_Cmd]  "Torque"
  Subsystem2/2(Pb_RF) -> [Braking_Pressure_RF]
  Gain9/1 -> [Vx_HV_mps]
  Gain10/1 -> [Vy_HV_mps]
  Gain3/1 -> [Ax_HV_mps2]
  Gain4/1 -> [Ay_HV_mps2]
  Gain22/1 -> Mux/1  "Driving_Torque_FL"
  Gain12/1 -> Mux/2  "Driving_Torque_FR"
  Zero-Order Hold8/1 -> MATLAB Function1/3(vx_th)
  Zero-Order Hold9/1 -> MATLAB Function1/4(ax)
  Zero-Order Hold10/1 -> MATLAB Function1/5(D_rel)
  Zero-Order Hold11/1 -> MATLAB Function1/6(V_rel)
  Zero-Order Hold12/1 -> MATLAB Function1/7(ax_rel)
  Zero-Order Hold13/1 -> MATLAB Function1/8(Qs)
  Zero-Order Hold14/1 -> MATLAB Function1/9(Rs)
  Abs/1 -> divide/1(dividend)
  Mux1/1 -> Scope11/1  "RR"
  [RR] -> Mux1/1  "RR"
  [RR_est] -> Mux1/2  "Est"
  [RVx] -> Mux2/1  "RV"
  [RV_est] -> Mux2/2  "Est"
  [RAx] -> Mux3/1  "RA"
  [RA_est] -> Mux3/2  "Est"
  Mux2/1 -> Scope11/2  "RV"
  Mux3/1 -> Scope11/3  "RA"
  [Braking_Pressure_RF] -> Gain36/1
  Gain33/1 -> Mux/3  "Driving_Torque_LF"
  [Braking_Pressure_LF] -> Gain33/1
  [Braking_Pressure_RL] -> Gain37/1
  Gain36/1 -> Mux/4  "Driving_Torque_RF"
  Gain38/1 -> Mux/6  "Driving_Torque_RR"
  Gain37/1 -> Mux/5  "Driving_Torque_RL"
  [Braking_Pressure_RR] -> Gain38/1
  [Braking_Pressure_LF] -> Scope12/1  "LF"
  [Braking_Pressure_RF] -> Scope12/2  "RF"
  [Braking_Pressure_RL] -> Scope12/3  "RL"
  [Braking_Pressure_RR] -> Scope12/4  "RR"
  MATLAB Function1/2(Y) -> Goto28/1  "MPC"
  Gain8/1 -> Scope18/1  "HV"
  Gain13/1 -> Scope18/2  "PV"
  [Vx_HV_mps] -> Acceleration controller2/2(Vxh)
  Zero-Order Hold17/1 -> Acceleration controller2/3(m)
  Zero-Order Hold18/1 -> Demux/1
  [RR] -> Scope13/2  "RR"
  Step/1 -> Scope2/1  "TH_limit"
  [TH] -> Scope2/2  "TH"
  Demux3/3 -> Zero-Order Hold12/1
  Zero-Order Hold3/1 -> MATLAB Function1/1(mode)
  [Driving_Torque] -> Gain22/1
  [Driving_Torque] -> Gain12/1
  [Vx_HV_mps] -> Gain8/1  "HV"
  [Vx_PV_mps] -> Gain13/1  "PV"
  Demux3/2 -> Zero-Order Hold11/1
  [Driving_Torque_Cmd] -> rolling_avg1/1(new_value)
  From16/1 -> MPC_ACC/3(Vx)
  From17/1 -> MPC_ACC/4(ax)
  Constant92/1 -> Zero-Order Hold1/1
  Constant5/1 -> Zero-Order Hold2/1
  Constant2/1 -> Subsystem/4(Ax_max)
  Constant6/1 -> Subsystem/5(Jx_max)
  From18/1 -> Subsystem/3(VehSpd)
  From21/1 -> MPC_ACC/2(vx_p)
  Subsystem/1("VREF_LongiVehSpdRef_mps ") -> Scope4/1  "mps"
  Zero-Order Hold1/1 -> MPC_ACC/5(Qs)
  Zero-Order Hold2/1 -> MPC_ACC/6(Rs)
  MATLAB Function1/1(u) -> cmd_limiter2/1(ax_cmd)  "cmd"
  From134/1 -> ?
  [ACCSetSpeed_mps] -> Mux5/10, Mux5/9, Mux5/8, Mux5/7, Mux5/6, Mux5/5, Mux5/4, Mux5/3, Mux5/2, Mux5/1
  Add Constant/1 -> Abs/1
  Constant11/1 -> Gain15/1
  Gain15/1 -> [ACCSetSpeed_mps]
  [ACCSetSpeed_mps] -> ACC_Mode_Selector/1(ACCSetSpeed_mps)
  [VACCTargetVehAssigned_flg] -> ACC_Mode_Selector/2(VACCTargetVehNotAssigned_flg)
  [Vx_HV_mps] -> ACC_Mode_Selector/4(Vx_HV_mps)
  [Vx_HV_mps] -> Gain20/1  "HV"
  Gain19/1 -> To Workspace7/1  "PV"
  Gain20/1 -> To Workspace6/1  "HV"
  Subsystem4/1(new_ave) -> Delay2/1, Delay2/2, Add10/2
  Add10/1 -> sample time1/1
  Delay2/1 -> Add10/1
  sample time1/1 -> Subsystem3/1(Jerk)  "Jerk"
  Step1/1 -> To Workspace9/1  "TH_limit"
  [Desired_distance] -> Scope13/1  "Desired_distance"
  [Desired_distance] -> Switch8/1, To Workspace12/1  "Desired_distance"
  Step2/1 -> Delay3/1
  Add11/1 -> To Workspace13/1, Delay/1
  Delay/1 -> Add11/2
  Delay3/1 -> Add11/1
  [Ax_HV_mps2] -> To Workspace14/1
  From103/1 -> Subsystem/2(VehSpd_Ref)
  [ACCSetSpeed_mps] -> Gain21/1
  Gain21/1 -> To Workspace15/1
  Mux5/1 -> [Vx_p]
  [Vx_HV_mps] -> 1-D Lookup Table Deccel Limit2/1
  1-D Lookup Table Deccel Limit2/1 -> To Workspace17/1
  [Vx_HV_mps] -> 1-D Lookup Table Accel Limit1/1
  1-D Lookup Table Accel Limit1/1 -> To Workspace16/1
  [Vx_HV_mps] -> 1-D Lookup Table Jerk UpLimit1/1
  [Vx_HV_mps] -> 1-D Lookup Table Jerk LowLimit1/1
  1-D Lookup Table Jerk UpLimit1/1 -> To Workspace18/1
  1-D Lookup Table Jerk LowLimit1/1 -> To Workspace19/1
  Demux3/1 -> Zero-Order Hold10/1  "Drel"
  [Acc_Mode] -> Logical Operator/1
  Constant29/1 -> divide/3(default_value)
  divide/1(quotient) -> Saturation1/1
  Saturation1/1 -> [TH]  "TH_default"
  Demux/7 -> [Station_HV_m]  "Station_HV"
  Constant9/1 -> Zero-Order Hold13/1
  Constant10/1 -> Zero-Order Hold14/1
  From39/1 -> Mux6/3
  From38/1 -> Mux6/2
  From31/1 -> Mux6/1
  Multiport Switch2/1 -> Demux3/1
  Mux6/1 -> Multiport Switch2/3
  Multiport Switch/1 -> Add Constant5/1, Add Constant/1
  Zero-Order Hold4/1 -> MPC_ACC/1(trig)
  Multiport Switch3/1 -> ACC_Mode_Selector/3(RR)
  [Acc_Mode] -> Scope6/1
  Smooth Switch/1(ax_cmd) -> Acceleration controller2/1(axc)
  Multiport Switch4/1 -> ACC_Mode_Selector/5(RV)
  [Vx_HV_mps] -> divide/2(divisor)
  Demux/8 -> [Steer_SW_deg]
  Demux/9 -> [Yaw_HV_deg]
  [X_HV_m] -> To Workspace/1
  [Y_HV_m] -> To Workspace1/1
  [Yaw_HV_deg] -> To Workspace2/1
  [Station_HV_m] -> To Workspace3/1
  [X_HV_m] -> global to local3/1(Xc)
  [Yaw_HV_deg] -> global to local3/3(Yaw)  "deg"
  [Y_HV_m] -> global to local3/2(Yc)
  Demux/10 -> Gain30/1
  Gain30/1 -> [Yaw_rate_radps]
  Constant26/1 -> MATLAB Function13/1(u)
  MATLAB Function13/1(y) -> XY Graph/1  "x"
  Constant27/1 -> MATLAB Function5/1(u)
  MATLAB Function5/1(y) -> XY Graph/2  "y"
  [X_HV_m] -> XY Graph/3  "X_HV"
  [Y_HV_m] -> XY Graph/4  "Y_HV"
  [Ay_HV_mps2] -> To Workspace24/1, Scope9/1
  sample time2/1 -> To Workspace4/1, Scope10/1  "Jerk"
  Delay6/1 -> Add4/1
  Add4/1 -> sample time2/1
  [Ay_HV_mps2] -> Add4/2, Delay6/2, Delay6/1
  [Vx_HV_mps] -> Switch5/2
  Switch5/1 -> To Workspace5/1
  Constant31/1 -> Switch5/1
  Constant33/1 -> Switch5/3
  Constant35/1 -> Switch6/3
  Constant34/1 -> Switch6/1
  Switch6/1 -> To Workspace21/1
  [Vx_HV_mps] -> Switch6/2
  Step3/1 -> Gain35/1, To Workspace22/1  "TH_limit"
  Gain35/1 -> To Workspace23/1
  [Steer_SW_deg] -> To Workspace26/1  "carsim"
  Demux/11 -> [y_error_m]
  [y_error_m] -> To Workspace25/1  "HV"
  Constant46/1 -> Manual Switch12/1
  Constant45/1 -> Manual Switch12/2
  Manual Switch12/1 -> ACCSpdCalculation/5(VDINR_ACCSpdResInc_flg)
  Manual Switch11/1 -> ACCSpdCalculation/4(VDINR_ACCSpdSetDec_flg)
  Constant24/1 -> Manual Switch11/2
  Constant39/1 -> Manual Switch11/1
  Manual Switch10/1 -> ACCSpdCalculation/3(NVDI_ACCSystemStatePrev_enum)
  Constant15/1 -> Manual Switch10/1
  Constant13/1 -> Manual Switch10/2
  Manual Switch/1 -> ACCSpdCalculation/2(NVDI_ACCActingPrev_flg)
  Constant12/1 -> Manual Switch/2
  Constant47/1 -> Manual Switch/1
  Switch1/1 -> [y_ref]
  [LeftDis_Camera] -> Switch1/1
  [LeftDis_PV] -> Switch1/3
  [LaneAvail_flg] -> Switch1/2  "LaneAvail_flg"
  [X_PV_m] -> XY Graph/5  "X_PV"
  [Y_PV_m] -> XY Graph/6  "Y_PV"
  cmd_limiter4/1(ax_cmd1) -> IC/1
  From163/1 -> ?
  Zero-Order Hold27/1 -> QP_logitudinal1/3(A_cons)
  MPC/3(M_act) -> Zero-Order Hold27/1
  Delay8/1 -> Mux9/4, MPC/7(ax_c_old), Goto31/1
  Zero-Order Hold26/1 -> QP_logitudinal1/2(f)
  MPC/4(gamma_act) -> Zero-Order Hold29/1
  From160/1 -> MPC/4(vxh)
  MPC/1(HH) -> Zero-Order Hold36/1
  From159/1 -> MPC/1(vx_p), MPC/2(vx_acc_set)
  Zero-Order Hold29/1 -> QP_logitudinal1/4(b)
  MPC/5(fesible_flag) -> Scope38/1
  Mux9/1 -> MPC/6(X_thk)
  Constant50/1 -> MPC/3(mode)
  MPC/2(ff) -> Zero-Order Hold26/1
  From245/1 -> QP_logitudinal1/5(u_old)
  Zero-Order Hold36/1 -> QP_logitudinal1/1(H)
  QP_logitudinal1/1(u) -> Scope21/1, Goto44/1, Delay8/1
  From149/1 -> Scope21/2  "ax_out"
  From161/1 -> MPC/5(axh)
  [spd_acc] -> Smooth Switch/1(Spd_acc_cmd)  "cmd"
  [Acc_Mode] -> Smooth Switch/2(Mode)
  [th_acc] -> Smooth Switch/3(TH_acc_cmd)  "cmd"
  MPC_ACC/1(u) -> cmd_limiter4/1(ax_cmd)  "cmd"
  [Vx_HV_mps] -> Subsystem3/2(Vx)
  Subsystem3/1(Out1) -> To Workspace8/1
  [TTC] -> Smooth Switch/4(TTC)
  global to local3/1(y_path_ref10) -> way2/1, Scope24/1
  Logical Operator/1 -> To Workspace20/1
  [Ax_HV_mps2] -> Subsystem4/1(new_value)
  Mux7/1 -> Multiport Switch2/2
  [RR] -> Switch8/3  "RR"
  Estimation_TTCx_PV2/2(TTC2) -> Switch13/3, Min/2
  Estimation_TTCx_PV2/1(TTC1) -> Min/1
  [RAx] -> Estimation_TTCx_PV2/3(A)
  Switch11/1 -> To Workspace10/1  "TH"
  [X_APV_m] -> To Workspace30/1
  [Station_APV_m] -> To Workspace36/1
  [Ax_APV_mps2] -> To Workspace34/1
  [Vx_APV_mps] -> Gain32/1
  [Y_APV_m] -> To Workspace31/1
  Gain32/1 -> To Workspace32/1
  Switch12/1 -> Cut-in strategy/3(TH)
  [Vx_HV_mps] -> Cut-in strategy/4(Vx_HV_mps)
  Cut-in strategy/1(TH*Vx) -> [RR_new], Scope32/1
  [Yaw_HV_deg] -> global to local2/3(Yaw)  "deg"
  [X_HV_m] -> global to local2/1(Xc)
  [Y_HV_m] -> global to local2/2(Yc)
  [X_PV_m] -> global to local2/4(X_ref)
  [Y_PV_m] -> global to local2/5(Y_ref)
  global to local2/1(x_ref) -> Scope78/2, [Rx]  "now"
  global to local2/2(y_ref) -> Scope77/2, [LeftDis_PV_one], [Ry]  "now"
  Add20/1 -> Mux14/2
  [Rx] -> Add20/1, Mux14/1
  From175/1 -> Add26/1, Scope30/1, Mux15/1
  Add26/1 -> Mux15/2
  Mux15/1 -> Goto95/1, Switch10/1, Scope36/1
  Mux14/1 -> Scope85/1, [x_translate]
  Switch10/1 -> descending/1, ascending/1
  From193/1 -> Switch9/2, Switch10/3
  descending/1 -> Switch9/3
  ascending/1 -> Switch9/1
  Switch9/1 -> 11:20/1, 1:10/1
  Manual Switch1/1 -> Goto93/1
  Constant67/1 -> [LaneAvail_flg]
  Demux/12 -> Gain57/1
  Gain57/1 -> Quantizer3/1
  Demux/13 -> Gain59/1
  Gain59/1 -> Quantizer4/1
  Demux/14 -> Gain60/1
  Gain60/1 -> Quantizer5/1
  Demux/15 -> Gain61/1
  Gain61/1 -> Quantizer6/1
  [Roll_rate_L1_radps] -> Add56/1
  [Roll_rate_L2_radps] -> Add56/2
  [Roll_rate_R1_radps] -> Add56/3
  [Roll_rate_R2_radps] -> Add56/4
  Add56/1 -> Gain/1
  Gain/1 -> rolling radius/1
  rolling radius/1 -> Gain56/1
  Gain43/1 -> To Workspace43/1  "est"
  From167/1 -> Gain43/1
  Gain40/1 -> To Workspace42/1  "carsim"
  From166/1 -> Gain40/1
  Constant19/1 -> [OnlyPY_signal]
  Constant38/1 -> Mux17/2
  Gain80/1 -> Vx5/2
  Kalman_Filter_LatSpd1/6(K) -> Display4/1, Scope23/1
  Gain55/1 -> Vx4/3  "small"
  From244/1 -> Gain55/1
  Compare To Constant2/1 -> Switch3/2
  Mux11/1 -> Kalman_Filter_LatSpd1/2(u)
  Kalman_Filter_LatSpd1/4(G) -> Display6/1
  Kalman_Filter_LatSpd1/7(M2) -> Delay48/1
  From257/1 -> Switch3/1
  From241/1 -> Kalman_Filter_LatSpd1/3(Yaw_rate)
  Kalman_Filter_LatSpd1/1(X_e) -> Delay49/1, Demux6/1
  Constant48/1 -> Kalman_Filter_LatSpd1/4(R)
  Constant44/1 -> Kalman_Filter_LatSpd1/5(Q)
  From242/1 -> Switch3/3
  Gain51/1 -> Vx6/1  "carsim"
  From258/1 -> Gain52/1
  Kalman_Filter_LatSpd1/3(F) -> Display5/1
  Demux8/1 -> Gain81/1
  From217/1 -> Scope41/1, Abs6/1
  From255/1 -> Gain54/1
  Gain81/1 -> Vx5/1
  Abs6/1 -> Compare To Constant2/1
  Demux8/2 -> Gain80/1
  Mux17/1 -> Delay49/2
  Demux6/2 -> Goto84/1
  Delay48/1 -> Kalman_Filter_LatSpd1/7(M)
  From247/1 -> Kalman_Filter_LatSpd1/6(y)
  Gain54/1 -> Vx4/2  "Est"
  Kalman_Filter_LatSpd1/2(X_k) -> Demux8/1
  Gain53/1 -> Vx4/1  "carsim"
  Gain52/1 -> Vx6/2  "est1"
  Kalman_Filter_LatSpd1/5(G2) -> Display7/1
  From232/1 -> Gain53/1
  From238/1 -> Gain51/1
  From243/1 -> Mux11/1
  From246/1 -> Mux11/2
  From248/1 -> Mux17/1
  Delay49/1 -> ?
  Demux6/1 -> Goto49/1
  [RR] -> Scope33/1  "RR"
  [RR_new] -> Scope33/2  "RR_new"
  Multiport Switch1/1 -> Cut-in strategy/5(RR)
  [Est_switch] -> Multiport Switch/1
  Constant/1 -> [Est_switch]
  [RR_est] -> Multiport Switch/3
  [Est_switch] -> Multiport Switch1/1
  [RR_est] -> Multiport Switch1/3
  [RR] -> Multiport Switch1/2
  From10/1 -> Multiport Switch2/1
  [Est_switch] -> Multiport Switch3/1
  [RR] -> Multiport Switch3/2
  [RR_est] -> Multiport Switch3/3
  [Est_switch] -> Multiport Switch4/1
  [RV_est] -> Multiport Switch4/3
  [RVx] -> Multiport Switch4/2
  Constant58/1 -> Zero-Order Hold3/1
  Constant54/1 -> LateralMotionKF1/8(lr)
  Gain44/1 -> LateralMotionKF1/4(delta)
  Constant56/1 -> LateralMotionKF1/1(T)
  From216/1 -> LateralMotionKF1/2(rk)
  From219/1 -> Unit Delay4/1
  From80/1 -> Display/1, LateralMotionKF1/3(vxk)
  Constant52/1 -> LateralMotionKF1/7(lf)
  Constant57/1 -> LateralMotionKF1/5(Caf)
  Constant59/1 -> LateralMotionKF1/6(Car)
  Constant55/1 -> LateralMotionKF1/9(mv)
  Unit Delay4/1 -> LateralMotionKF1/10(vyk)
  From221/1 -> Gain41/1  "carsim"
  Gain41/1 -> Gain44/1  "deg"
  From233/1 -> Scope50/1
  LateralMotionKF1/1(vyk1) -> Goto90/1, Scope50/2
  1:10/1 -> Manual Switch1/1
  11:20/1 -> Manual Switch1/2
  From234/1 -> Unit Delay5/1
  Unit Delay5/1 -> Mux10/2
  From237/1 -> Delay10/2
  Delay10/1 -> Mux10/1
  From239/1 -> Delay10/1
  Mux10/1 -> Kalman_Filter_LatSpd1/1("X_e ")
  Constant61/1 -> Switch2/3
  Relational Operator3/1 -> Switch2/2
  From253/1 -> Relational Operator3/1
  Constant60/1 -> Relational Operator3/2
  Switch3/1 -> Switch2/1
  Switch2/1 -> Goto91/1
  Multiport Switch5/1 -> [LeftDis_PV]
  Constant62/1 -> Multiport Switch5/1
  [LeftDis_PV_one] -> Multiport Switch5/2
  [LeftDis_PV_multi] -> Multiport Switch5/3
  Mux16/1 -> [yaw_rotate]
  Add62/1 -> Delay50/1, Gain72/1
  T/1 -> Add62/1
  Delay50/1 -> Add62/2
  r/l/1 -> Scope16/2, T/1  "yaw_rate_est"
  Add60/1 -> r/l/1
  [Roll_rate_R1_radps] -> Add60/2
  [Roll_rate_L1_radps] -> Add60/1
  From273/1 -> Reshape/1
  Reshape/1 -> Gain46/1
  Gain42/1 -> Cos/1
  Cos/1 -> Product2/2
  Product2/1 -> [delta_y_19]
  [Ry] -> Add32/1, Mux20/1
  Add32/1 -> Mux20/2
  Mux20/1 -> [y_translate]
  [Vx_HV_mps] -> Gain45/1
  record_delta_x/1(delta_x_19) -> [delta_x_19]
  Gain56/1 -> record_delta_x/1(delta_x)
  From188/1 -> Switch10/2
  [delta_x_19] -> Product2/1
  Gain46/1 -> Subsystem6/1(delta__y)
  Subsystem6/1(delta__y_19) -> Add26/2
  Constant63/1 -> Mux16/1
  [delta_yaw] -> Mux16/2
  [delta_yaw] -> Gain42/1
  record_delta_yaw/1(delta_yaw_19) -> Scope56/1, [delta_yaw]
  Gain72/1 -> To Workspace40/1, Scope5/2, record_delta_yaw/1(delta_yaw)  "yaw_est"
  [delta_y_19] -> Add32/2
  [delta_x_19] -> Add20/2
  [Yaw_HV_deg] -> Scope5/1  "carsim"
  [Yaw_rate_radps] -> Scope16/1  "carsim"
  [Station_HV_m] -> preview/1(In1)
  [Vx_HV_mps] -> preview/2(In2)
  preview/1(X_ref) -> global to local3/4(X_ref)
  preview/2(Y_ref) -> global to local3/5(Y_ref)
  PV_trajectory_planning/1(LeftDis_PV_multi) -> [LeftDis_PV_multi], Scope58/1
  [x_translate] -> PV_trajectory_planning/1(x_translate)
  [yaw_rotate] -> PV_trajectory_planning/2(yaw_rotate)
  [y_translate] -> PV_trajectory_planning/3(y_translate)
  [Ry] -> PV_trajectory_planning/4(Ry)
  Demux/16 -> Add Constant4/1  "dist_acc"
  Demux/18 -> Gain47/1
  Demux/23 -> [X_PV_m]  "X_Obj_1"
  Demux/17 -> [VACCTargetVehAssigned_flg]  "DisS1_1"
  Demux/21 -> Gain48/1
  Demux/20 -> [sensor_dectect_y_m]
  Demux/19 -> [sensor_dectect_x_m]
  Demux/24 -> [Y_PV_m]  "Y_Obj_1"
  Add Constant4/1 -> [Desired_distance_carsim_m]
  Gain47/1 -> [sensor_dectect_spd_mps]
  Gain48/1 -> [sensor_dectect_Vx_mps]
  Demux/22 -> Gain49/1
  Gain49/1 -> [sensor_dectect_Vy_mps]
  Demux/25 -> Gain58/1
  Demux/26 -> Gain50/1
  Gain50/1 -> [Ax_PV_mps2]
  Gain58/1 -> [Vx_PV_mps]
  Demux/27 -> [Station_PV_m]
  Demux/32 -> [Station_APV_m]
  Demux/28 -> [X_APV_m]  "X_Obj_3"
  Demux/29 -> [Y_APV_m]  "Y_Obj_3"
  Demux/30 -> Gain1/1
  Gain1/1 -> [Vx_APV_mps]
  Demux/31 -> [Ax_APV_mps2]
  Constant28/1 -> Zero-Order Hold4/1
  From212/1 -> Mux7/1  "RR"
  [Vx_HV_mps] -> divide2/2(divisor)
  Saturation7/1 -> [TH_plot]  "TH_default"
  divide2/1(quotient) -> Saturation7/1
  Constant7/1 -> divide2/3(default_value)
  Add Constant5/1 -> Abs4/1
  Abs4/1 -> divide2/1(dividend)
  [RR] -> Estimation_TTCx_PV2/1(R)
  [TTC] -> Cut-in strategy/2(TTC)
  From49/1 -> Mux7/2
  [RVx] -> Estimation_TTCx_PV2/2(V)
  Constant20/1 -> divide3/3(default_value)
  Saturation/1 -> Abs2/1
  [Acc_Mode] -> Switch8/2
  Switch8/1 -> To Workspace11/1
  [Acc_Mode] -> Switch11/2
  [TH_plot] -> Switch11/3  "TH"
  Constant22/1 -> Switch11/1
  V_rel Estimation/1(s_rel) -> [RR_est]
  V_rel Estimation/2(v_rel) -> [RV_est]
  V_rel Estimation/3(a_rel) -> [RA_est]
  [RR] -> Mux4/1
  [Ax_HV_mps2] -> V_rel Estimation/2(a_c)
  [RVx] -> Mux4/2
  [RR] -> V_rel Estimation/3(S_rel)
  [cut_in_flg] -> V_rel Estimation/1(cut_in_flg)
  Mux4/1 -> V_rel Estimation/4(initial_value)
  [RAx] -> Mux4/3
  [VACCTargetVehAssigned_flg] -> Switch12/2
  [Vx_PV_mps] -> Gain19/1  "PV"
  Constant8/1 -> Subsystem/1("Trig ")
  [RR] -> Multiport Switch/2
  IC/1 -> Goto24/1
  Switch13/1 -> Scope7/1, [TTC]
  [RR] -> divide3/1(dividend)
  Abs2/1 -> Compare To Constant5/1, Detect Increase/1
  Detect Increase/1 -> Logical Operator3/1
  [TTC_Increase_flg] -> Cut-in strategy/1(TTC_Increase_flg)
  divide3/1(quotient) -> Saturation/1
  Logical Operator3/1 -> [TTC_Increase_flg]
  Compare To Constant5/1 -> Logical Operator3/2
  [RR] -> Compare To Constant4/1
  Compare To Constant4/1 -> Switch13/2
  Constant21/1 -> Switch13/1
  Delay1/1 -> Add15/2
  [Yaw_rate_radps] -> Scope70/1  "carsim"
  Add9/1 -> r/l1/1
  Add15/1 -> Delay1/1, Gain5/1
  [Yaw_HV_deg] -> Scope71/1  "carsim"
  [Roll_rate_R1_radps] -> Scope72/2, Quantizer2/1
  [Roll_rate_L1_radps] -> Quantizer1/1
  T1/1 -> Add15/1
  Gain5/1 -> Scope71/2  "yaw_est"
  r/l1/1 -> Scope70/2, T1/1  "yaw_rate_est"
  Quantizer1/1 -> Add9/1
  Quantizer2/1 -> Scope72/1, Add9/2
  Quantizer3/1 -> [Roll_rate_L1_radps]
  Quantizer6/1 -> [Roll_rate_R2_radps]
  Quantizer5/1 -> [Roll_rate_R1_radps]
  Quantizer4/1 -> [Roll_rate_L2_radps]
  Mux/1 -> CarSim S-Function/1
  [Desired_distance] -> Scope75/1  "Desired_distance"
  From50/1 -> Scope76/1, Mux7/3
  [RR] -> Scope75/2
  Constant23/1 -> Switch12/3
  [TH] -> Switch12/1
  Camera/1(LeftDis) -> [LeftDis_Camera]
  [Yaw_HV_deg] -> Camera/2(deg)  "deg"
  [Ax_HV_mps2] -> Camera/6(Ax_HV_mps2)
  [Y_HV_m] -> Camera/4(Yo)
  [Vx_HV_mps] -> Camera/1(mps)  "mps"
  [X_HV_m] -> Camera/3(Xo)
  [Station_HV_m] -> Camera/5(station)
  [Est_switch] -> V_rel Estimation/Enable
  Zero-Order Hold23/1 -> MPC_Bicycle_LDC1/3(Qs)
  From155/1 -> MPC_Bicycle_LDC1/9(Ax)
  Zero-Order Hold5/1 -> MPC_Bicycle_LDC1/1(trig)
  Zero-Order Hold24/1 -> MPC_Bicycle_LDC1/4(Rs)
  From129/1 -> Scope3/1, Demux2/1
  [Vx_HV_mps] -> Gain31/1
  From176/1 -> MATLAB Function17/7(Vx)
  Gain14/1 -> MATLAB Function17/6(steer_angle)
  Subsystem17/1(new_ave) -> [Steer_IN_deg]
  Demux2/1 -> MPC_Bicycle_LDC1/2(Yref)
  [Steer_Dynamic_deg] -> Smooth Switch1/1(Dynamic_cmd)
  Radians to Degrees2/1 -> Gain28/1
  From23/1 -> Scope1/2
  From153/1 -> MPC_Bicycle_LDC1/5(Vy)
  Relational Operator/1 -> Latch/1(set)
  Constant30/1 -> Relational Operator/2
  From174/1 -> Mux8/3  "carsim"
  From214/1 -> R selector/1(In1)
  Delay4/1 -> Gain24/1
  [Steer_Kinematic_deg] -> Smooth Switch1/3(Kinematic_cmd)
  From128/1 -> Gain26/1  "carsim"
  Relational Operator2/1 -> Switch/2
  From177/1 -> MATLAB Function17/8(Ax)
  Switch/1 -> Radians to Degrees1/1, Unit Delay/1
  From92/1 -> 1-D Lookup Table1/1
  Unit Delay/1 -> Switch/1
  Constant16/1 -> Zero-Order Hold19/1
  Zero-Order Hold19/1 -> MATLAB Function17/1(trig)
  Delay7/1 -> Gain25/1
  Smooth Switch1/1(ax_cmd) -> Subsystem17/1(new_value)
  R selector/1(Out1) -> Zero-Order Hold22/1
  From25/1 -> Gain34/1  "carsim"
  Gain28/1 -> Saturation4/1  "deg"
  From164/1 -> 1-D Lookup Table2/1
  From24/1 -> R selector/2(vx)
  Gain27/1 -> MPC_Bicycle_LDC1/7(steer_angel)
  Gain31/1 -> Relational Operator/1, Relational Operator1/1  "kph"
  From154/1 -> Subsystem1/1(In1)
  Saturation4/1 -> Goto38/1, Scope25/1, Goto127/1, Delay7/1  "mpc"
  Switch4/1 -> Unit Delay2/1, Radians to Degrees2/1
  Latch/1(latched) -> Smooth Switch1/2(Mode), [LFC_Mode]
  MATLAB Function17/1(u) -> Relational Operator2/1, Switch/3
  From170/1 -> R selector1/1(In1)
  Unit Delay2/1 -> Switch4/1
  1-D Lookup Table2/1 -> Zero-Order Hold21/1
  From173/1 -> MATLAB Function17/2(Yref)
  Radians to Degrees1/1 -> Gain23/1
  Zero-Order Hold22/1 -> MATLAB Function17/5(Rs)
  MPC_Bicycle_LDC1/1(u) -> Switch4/3, Relational Operator4/1
  Gain34/1 -> Manual Switch5/1  "deg"
  Mux8/1 -> Scope1/1
  Gain24/1 -> Manual Switch5/2  "deg"
  Manual Switch9/1 -> Gain27/1
  Manual Switch5/1 -> Gain14/1
  Saturation3/1 -> Goto128/1, Mux8/2, Goto19/1, Delay4/1  "Kinematic"
  Constant17/1 -> Zero-Order Hold20/1
  From169/1 -> R selector1/2(vx)
  Gain23/1 -> Saturation3/1  "deg"
  From126/1 -> Mux8/1  "Dynamic"
  Gain25/1 -> Manual Switch9/2  "deg"
  Relational Operator4/1 -> Switch4/2
  Constant42/1 -> Zero-Order Hold24/1
  Gain26/1 -> Manual Switch9/1  "deg"
  From127/1 -> MPC_Bicycle_LDC1/6(yaw_rate)
  Zero-Order Hold20/1 -> MATLAB Function17/3(tau)
  Zero-Order Hold21/1 -> MATLAB Function17/4(Qs)
  Subsystem1/1(Out1) -> MPC_Bicycle_LDC1/8(Vx)
  From162/1 -> Scope25/2  "carsim"
  Relational Operator1/1 -> Latch/2(reset)
  Constant32/1 -> Relational Operator1/2
  Constant3/1 -> Zero-Order Hold5/1
  1-D Lookup Table1/1 -> Scope/1, Zero-Order Hold23/1
  Constant51/1 -> Subsystem8/11(TH_trig)
  From192/1 -> Subsystem8/6(RV_est)
  From187/1 -> Subsystem8/5(RR_est)
  From199/1 -> Subsystem8/10(Ax_HV_mps2)
  From268/1 -> Subsystem8/4(RAx)
  From185/1 -> Subsystem8/2(RR_new)  "RR"
  From195/1 -> Subsystem8/7(RA_est)
  Subsystem8/2(Desired_distance) -> Goto40/1
  From181/1 -> Subsystem8/1(Est_switch)
  Subsystem8/1(th_acc) -> Goto39/1
  From200/1 -> Subsystem8/3(RVx)
  From191/1 -> Subsystem8/9(Vx_HV_mps)
  From190/1 -> Subsystem8/8(ACCSetSpeed_mps)
  From186/1 -> MATLAB Function1/2(ACCSetSpeed_mps)
  Subsystem8/3(spd_acc) -> Goto41/1
  From55/1 -> Subsystem8/12(vx_p)
  Constant83/1 -> rolling_avg1/4(tc)
  rolling_avg1/1(new_ave) -> [Driving_Torque], Delay11/1
  Delay11/1 -> rolling_avg1/2(old_ave)
  Constant84/1 -> rolling_avg1/3(delta_t)  "T"
  [Steer_IN_deg] -> Mux/7
  [sensor_dectect_x_m] -> Scope78/1
  [sensor_dectect_y_m] -> Scope77/1
  From402/1 -> Subsystem5/5(yaw_rate)
  From397/1 -> Subsystem5/1(Yref)
  From403/1 -> Subsystem5/6(Vy)
  From396/1 -> Subsystem5/2(vx)
  From401/1 -> Subsystem5/4(Ax)
  Constant85/1 -> Subsystem5/Enable
  From399/1 -> Subsystem5/3(carsim)  "carsim"
  From398/1 -> Subsystem5/7(LaneAvail_flg)  "LaneAvail_flg"
  Subsystem5/1(Out3) -> Goto126/1
  MATLAB Function17/2(F) -> Scope84/1, Display1/1
  Cos1/1 -> Product3/2
  From437/1 -> Multiport Switch10/2
  From435/1 -> Gain73/1
  Add19/1 -> Mux25/2
  Add23/1 -> Delay14/1, Gain75/1
  record_delta_x1/1(delta_x_19) -> Goto144/1
  From448/1 -> global to local1/4(X_ref)
  PV_trajectory_planning1/1(LeftDis_PV_multi) -> Goto142/1, Scope89/1
  Add22/1 -> r/l2/1
  record_delta_yaw1/1(delta_yaw_19) -> Scope88/1, Goto133/1
  Gain71/1 -> Cos1/1
  From455/1 -> PV_trajectory_planning1/2(yaw_rotate)
  From429/1 -> Switch15/1
  From446/1 -> Scope87/1  "carsim"
  From433/1 -> Switch15/2  "LaneAvail_flg"
  Product3/1 -> Goto134/1
  From447/1 -> Scope86/1  "carsim"
  r/l2/1 -> Scope86/2, T2/1  "yaw_rate_est"
  Delay14/1 -> Add23/2
  Constant98/1 -> Multiport Switch10/1
  From438/1 -> Multiport Switch10/3
  Multiport Switch10/1 -> Goto136/1
  Mux24/1 -> Goto141/1
  T2/1 -> Add23/1
  Gain74/1 -> record_delta_x1/1(delta_x)
  From445/1 -> Add7/2
  Mux25/1 -> Goto143/1
  global to local1/1(x_ref) -> Scope91/2, Goto138/1  "now"
  From440/1 -> Gain71/1
  Mux23/1 -> Scope92/1, Goto140/1
  From431/1 -> Mux24/2
  From452/1 -> Add21/3
  From430/1 -> Switch15/3
  Switch15/1 -> Goto135/1
  From436/1 -> Product3/1
  From441/1 -> global to local1/1(Xc)
  From444/1 -> global to local1/3(Yaw)  "deg"
  Add7/1 -> Mux23/2
  From432/1 -> Add7/1, Mux23/1
  Constant99/1 -> Mux24/1
  From451/1 -> PV_trajectory_planning1/3(y_translate)
  From450/1 -> Add21/2
  From443/1 -> global to local1/2(Yc)
  Gain75/1 -> To Workspace27/1, Scope87/2, record_delta_yaw1/1(delta_yaw)  "yaw_est"
  From456/1 -> PV_trajectory_planning1/4(Ry)
  From449/1 -> global to local1/5(Y_ref)
  From458/1 -> Add22/2
  global to local1/2(y_ref) -> Scope90/2, Goto137/1, Goto139/1  "now"
  From454/1 -> PV_trajectory_planning1/1(x_translate)
  rolling radius1/1 -> Gain74/1
  From442/1 -> Add19/2
  Gain70/1 -> rolling radius1/1
  From453/1 -> Add21/4
  From439/1 -> Add21/1
  From459/1 -> Scope90/1
  From457/1 -> Add22/1
  From434/1 -> Add19/1, Mux25/1
  Add21/1 -> Gain70/1
  [RVx] -> Multiport Switch14/2
  [RV_est] -> Multiport Switch14/3
  [Est_switch] -> Multiport Switch14/1
  [RR_est] -> Multiport Switch13/3
  [RR] -> Multiport Switch13/2
  [Est_switch] -> Multiport Switch13/1
  Multiport Switch14/1 -> ACC_Mode_Selector3/5(RV)
  Multiport Switch13/1 -> ACC_Mode_Selector3/3(RR)
  [Vx_HV_mps] -> ACC_Mode_Selector3/4(Vx_HV_mps)
  [VACCTargetVehAssigned_flg] -> ACC_Mode_Selector3/2(VACCTargetVehNotAssigned_flg)
  [ACCSetSpeed_mps] -> ACC_Mode_Selector3/1(ACCSetSpeed_mps)
  MPC_ACC5/1(A) -> Subsystem21/1(A)  "cmd"
  MPC_ACC5/2(B) -> Subsystem21/2(B)
  MPC_ACC5/3(C) -> Subsystem21/3(C)
  MPC_ACC5/4(Yref) -> Subsystem21/4(Yref)
  MPC_ACC5/5(x_state) -> Subsystem21/5(x_state)
  Subsystem21/1(cmd) -> [delta_u_Spd], cmd_limiter9/1(ax_cmd)
  cmd_limiter9/1(ax_cmd1) -> [spd_acc]
  [Vx_p] -> MPC_ACC5/1(vx_p)
  [Vx_HV_mps] -> MPC_ACC5/2(Vx)
  [Vx_HV_mps] -> MPC_ACC4/4(vx)
  cmd_limiter11/1(ax_cmd1) -> [th_acc]
  MPC_ACC4/5(x_state) -> Subsystem23/5(x_state)
  MPC_ACC4/4(Yref) -> Subsystem23/4(Yref)
  MPC_ACC4/3(C) -> Subsystem23/3(C)
  MPC_ACC4/2(B) -> Subsystem23/2(B)
  MPC_ACC4/1(A) -> Subsystem23/1(A)  "cmd"
  [RR_new] -> MPC_ACC4/1(D_rel)  "RR"
  [ACCSetSpeed_mps] -> MPC_ACC4/5(ACCSetSpeed_mps)
  [RVx] -> MPC_ACC4/2(V_rel)
  [Ax_HV_mps2] -> MPC_ACC5/3(ax)
  [Ax_HV_mps2] -> MPC_ACC4/6(ax)
  [Ax_HV_mps2] -> Add25/1
  [RAx] -> Add25/2
  Add25/1 -> cmd_limiter11/1(ax_cmd)
  Constant104/1 -> Subsystem22/11(TH_trig)
  From512/1 -> Subsystem22/6(RV_est)
  From509/1 -> Subsystem22/5(RR_est)
  From514/1 -> Subsystem22/10(Ax_HV_mps2)
  From516/1 -> Subsystem22/4(RAx)
  From508/1 -> Subsystem22/2(RR_new)  "RR"
  From513/1 -> Subsystem22/7(RA_est)
  Subsystem22/2(Desired_distance) -> Goto153/1
  From507/1 -> Subsystem22/1(Est_switch)
  Subsystem22/1(th_acc) -> Goto152/1
  From515/1 -> Subsystem22/3(RVx)
  From511/1 -> Subsystem22/9(Vx_HV_mps)
  From510/1 -> Subsystem22/8(ACCSetSpeed_mps)
  Subsystem22/3(spd_acc) -> Goto155/1
  From517/1 -> Subsystem22/12(vx_p)
  [ax] -> Subsystem23/6(u_old)
  [Acc_Mode] -> Smooth Switch4/2(Mode)
  Delay17/1 -> Smooth Switch4/1(Spd_acc_cmd)
  Delay18/1 -> Smooth Switch4/3(TH_acc_cmd)
  Smooth Switch4/1(ax_cmd) -> cmd_limiter1/1(ax_cmd)
  [ax] -> Subsystem21/6(u_old)
  MPC_ACC4/6(Desired_dist) -> [Desired_distance]
  Compare To Zero/1 -> Steer_Kinematic/Enable
  [Vx_HV_mps] -> Gain78/1
  Delay19/1 -> [delta_u_K]
  [Vx_HV_mps] -> 1-D Lookup Table7/1
  Dynamic_Model/5(x_state) -> Bus Creator/5
  Dynamic_Model/4(Yref) -> Bus Creator/4
  Subsystem25/1(rad) -> Dynamic_Model/3(steer_angle)
  1-D Lookup Table8/1 -> Steer_Kinematic/2(Q)
  [Vy_HV_mps] -> Dynamic_Model/4(Vy)
  [LaneAvail_flg] -> R selector4/1(LaneAvail_fig)
  Delay16/1 -> [delta_u_D]
  Compare To Zero1/1 -> Steer_Dynamic/Enable
  R selector5/1(R_D) -> Steer_Dynamic/3(R)
  Gain82/1 -> Gain79/1  "deg"
  [u_old] -> Steer_Kinematic/4(u_old)
  [Vx_HV_mps] -> Dynamic_Model/1(vx)
  R selector4/1(R) -> Steer_Kinematic/3(R)
  1-D Lookup Table7/1 -> Gain6/1
  Kinematic_Model/3(C) -> Bus Creator1/3
  Bus Creator1/1 -> Steer_Kinematic/1(Model)
  [LaneAvail_flg] -> R selector5/1(LaneAvail_flg)
  Gain78/1 -> Relational Operator10/1, Relational Operator9/1  "kph"
  Latch2/1(latched) -> Switch16/2
  Constant106/1 -> Relational Operator9/2
  Relational Operator10/1 -> Latch2/2(reset)
  Kinematic_Model/1(A) -> Bus Creator1/1
  Kinematic_Model/5(x_state) -> Bus Creator1/5
  Limit/1 -> [Steer_Kinematic_deg]
  [Vx_HV_mps] -> 1-D Lookup Table8/1
  Kinematic_Model/4(Yref) -> Bus Creator1/4
  [y_ref] -> Kinematic_Model/2(Yref_K)
  [Vx_HV_mps] -> R selector5/2(vx)
  Constant107/1 -> Relational Operator10/2
  Switch16/1 -> [u_old]
  Gain79/1 -> Kinematic_Model/3(steer_angle)
  Relational Operator9/1 -> Latch2/1(set)
  Constant105/1 -> Limit1/3
  [u_old] -> Steer_Dynamic/4(u_old)
  Radians to Degrees5/1 -> Gain77/1
  Gain77/1 -> Limit1/1  "deg"
  Constant101/1 -> Limit1/2
  Steer_Dynamic/1(cmd) -> Radians to Degrees5/1, Delay16/1
  [Steer_SW_deg] -> Subsystem25/1(carsim)  "carsim"
  Limit1/1 -> [Steer_Dynamic_deg]
  Dynamic_Model/3(C) -> Bus Creator/3
  Dynamic_Model/1(A) -> Bus Creator/1
  Bus Creator/1 -> Steer_Dynamic/1(Model)
  Dynamic_Model/2(B) -> Bus Creator/2
  Steer_Kinematic/1(cmd) -> Radians to Degrees6/1, Delay19/1
  [Vx_HV_mps] -> R selector4/2(vx)
  [Steer_SW_deg] -> Gain82/1  "carsim"
  [Vx_HV_mps] -> Kinematic_Model/1(vx)
  Radians to Degrees6/1 -> Gain83/1
  Constant102/1 -> Limit/2
  Gain83/1 -> Limit/1  "deg"
  Constant103/1 -> Limit/3
  [Yaw_rate_radps] -> Dynamic_Model/5(yaw_rate)
  Kinematic_Model/2(B) -> Bus Creator1/2
  [Y_PV_m] -> Relative_Dynamic/2(Y_PV_m)
  Relative_Dynamic/3(RA) -> [RAx]
  Relative_Dynamic/2(RV) -> [RVx]
  [X_APV_m] -> Relative_Dynamic/5(X_APV_m)
  Relative_Dynamic/4(trig) -> [cut_in_flg]
  [Y_APV_m] -> Relative_Dynamic/6(Y_APV_m)
  [ACCSetSpeed_mps] -> Relative_Dynamic/12(ACCSetSpeed_mps)
  [VACCTargetVehAssigned_flg] -> Relative_Dynamic/14(VACCTargetVehAssigned_flg)
  [Ax_APV_mps2] -> Relative_Dynamic/13(Ax_APV_mps2)  "PV"
  [OnlyPY_signal] -> Relative_Dynamic/15(OnlyPV_signal)
  [X_HV_m] -> Relative_Dynamic/3(X_HV_m)
  [X_PV_m] -> Relative_Dynamic/1(X_PV_m)
  [Y_HV_m] -> Relative_Dynamic/4(Y_HV_m)
  [Vx_HV_mps] -> Relative_Dynamic/8(Vx_HV_mps)
  [Ax_PV_mps2] -> Relative_Dynamic/9(Ax_PV_mps2)  "PV"
  [Vx_APV_mps] -> Relative_Dynamic/11(Vx_APV_mps)
  [Vx_PV_mps] -> Relative_Dynamic/7(Vx_PV_mps)
  Relative_Dynamic/1(RR) -> [RR]
  [Ax_HV_mps2] -> Relative_Dynamic/10(Ax_HV_mps2)  "HV"
  [TTC] -> To Workspace29/1
  [RVx] -> divide3/2(divisor)
  cmd_limiter1/1(ax_cmd1) -> [ax]
  [Acc_Mode] -> Subsystem21/Enable
  [Acc_Mode] -> Logical Operator1/1
  Logical Operator1/1 -> Subsystem23/Enable
  ACC_Mode_Selector3/1(Out1) -> [Acc_Mode]
  cmd_limiter2/1(ax_cmd1) -> Goto22/1
  [delta_u_TH] -> Delay18/1
  [delta_u_Spd] -> Delay17/1
  [LFC_Mode] -> Compare To Zero/1
  [LFC_Mode] -> Compare To Zero1/1
  [y_ref] -> Dynamic_Model/2(Yref_D)
  ACC_Mode_Selector/1(Out1) -> Goto30/1
  [delta_u_K] -> Switch16/3
  [delta_u_D] -> Switch16/1
  Gain6/1 -> Steer_Dynamic/2(Q)
  Subsystem23/1(cmd) -> Add25/3, [delta_u_TH]
  [RAx] -> MPC_ACC4/3(ax_rel)
  From137/1 -> MPC_ACC1/3(ax_rel)
  Subsystem7/1(cmd) -> Goto58/1, Add1/3
  Logical Operator2/1 -> Subsystem7/Enable
  MPC_ACC1/6(Desired_dist) -> Goto50/1
  From142/1 -> Subsystem7/6(u_old)
  Add1/1 -> cmd_limiter3/1(ax_cmd)
  From141/1 -> Add1/2
  From140/1 -> Add1/1
  From139/1 -> MPC_ACC1/6(ax)
  From135/1 -> MPC_ACC1/2(V_rel)
  From138/1 -> MPC_ACC1/5(ACCSetSpeed_mps)
  From124/1 -> MPC_ACC1/1(D_rel)  "RR"
  MPC_ACC1/1(A) -> Subsystem7/1(A)  "cmd"
  MPC_ACC1/2(B) -> Subsystem7/2(B)
  MPC_ACC1/3(C) -> Subsystem7/3(C)
  MPC_ACC1/4(Yref) -> Subsystem7/4(Yref)
  MPC_ACC1/5(x_state) -> Subsystem7/5(x_state)
  cmd_limiter3/1(ax_cmd1) -> Goto54/1
  From132/1 -> MPC_ACC1/4(vx)
